simulink model "speedgoat_IO397_RCP"  (R2022b)
settings: Solver=FixedStepDiscrete  StartTime=0.0  StopTime=inf  RelTol=1e-3
PreLoadFcn:
  | Ts = 0.001;
  | FPGA_Frequency = 75000000;
undefined symbols (not defined in the file): IO397
libraries: speedgoatlib_fpga_dio x2, speedgoatlib_fpga_analog_io x2, speedgoatlib_fpga_inta x1, simulink x1, speedgoatlib_interrupt x1, speedgoatlib_fpga_pwm x1, speedgoatlib_fpga_quadrature x1, speedgoatlib_fpga x1
settings Model: SimulationMode=external  Creator=simon.beck  LastModifiedBy=jeffrey.gruenig
settings SolverCC: ConcurrentTasks=on  PositivePriorityOrder=on  MaxZcPerStep=1
settings DataIOCC: SaveFormat=StructureWithTime
settings OptimizationCC: BlockReduction=off  OptimizeBlockIOStorage=off  BufferReuse=off
settings DebuggingCC: UnderspecifiedInitializationDetection=Classic  MergeDetectMultiDrivingBlocksExec=none  TasksWithSamePriorityMsg=none
settings HardwareCC: ProdBitPerLong=64  ProdLongLongMode=on  ProdHWDeviceType=Intel->x86-64 (Linux 64)
settings ModelReferenceCC: EnableRefExpFcnMdlSchedulingChecks=on  PropagateSignalLabelsOutOfModel=off
settings RTWCC: Description=Simulink Real-Time  SystemTargetFile=slrealtime.tlc  TemplateMakefile=slrealtime_default_tmf  Toolchain=Simulink Real-Time Toolchain  BuildConfiguration=Faster Runs  CodeExecutionProfiling=on  TargetLang=C++  DLArmComputeVersion=19.05

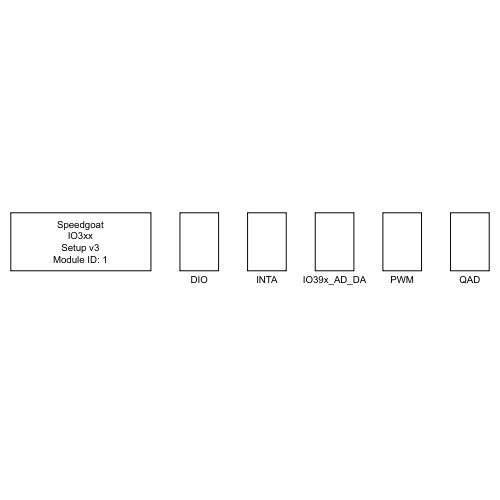
[thumbnail: Simulink's stored preview of the top-level diagram]
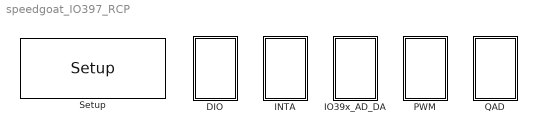
== system speedgoat_IO397_RCP ==
  DIO : Subsystem
  INTA : Subsystem
  IO39x_AD_DA : Subsystem
  PWM : Subsystem
  QAD : Subsystem
  Setup : speedgoatlib_fpga/Setup/Setup  board=IO397-50k  id=1  device_id=1  frontIO=None  rearIO=None  bitstreamFile=speedgoat_IO397_RCP.mat  rev=6.100000  timestamp_string=06/12/23 16:45:41  fpgaFreq=75 MHz  fpgaTick=13.33 ns  ProgSpiFlash=off  ProgBPIFlash=off  pciSlot=-1  useFpgaDmaController=off  PullRPort0=pull-up 3.3V  VioPort0=3.3V  PullRPort1=pull-up 3.3V  VioPort1=3.3V  PullRPort2=pull-up 3.3V  VioPort2=3.3V  PullRPort3=pull-up 3.3V  VioPort3=3.3V  PullRPort4=pull-up 3.3V  VioPort4=3.3V  PullRPort5=pull-up 3.3V  VioPort5=3.3V  PullRPort6=pull-up 3.3V  VioPort6=3.3V  diffLineTermination_rear1=on  diffLineTermination_rear2=on  diffLineTermination_rear3=on  diffLineTermination_rear4=on  diffLineTermination_rear5=on  diffLineTermination_rear6=on  diffLineTermination_rear7=on  diffLineTermination_rear8=on  PullRPort15=pull-up 3.3V  PullRPort31=pull-up 3.3V  PullRPort47=pull-up 3.3V  PullRPort63=pull-up 3.3V  diffLineTermination_1=on  diffLineTermination_2=on  diffLineTermination_3=on  diffLineTermination_4=on  diffLineTermination_5=on  diffLineTermination_6=on  diffLineTermination_7=on  diffLineTermination_8=on  diffLineTermination_9=on  diffLineTermination_10=on  diffLineTermination_11=on  diffLineTermination_12=on  diffLineTermination_13=on  diffLineTermination_14=on  diffLineTermination_15=on  diffLineTermination_16=on  diffLineTermination_17=on  diffLineTermination_18=on  diffLineTermination_19=on  diffLineTermination_20=on  diffLineTermination_21=on  diffLineTermination_22=on  diffLineTermination_23=on  diffLineTermination_24=on  diffLineTermination_25=on  diffLineTermination_26=on  diffLineTermination_27=on  diffLineTermination_28=on  diffLineTermination_29=on  diffLineTermination_30=on  diffLineTermination_31=on  diffLineTermination_32=on  Vo_36x_1=3.3V  Vi_Pull_36x_1=Floating  Vo_36x_2=3.3V  Vi_Pull_36x_2=Floating  Vo_36x_3=3.3V  Vi_Pull_36x_3=Floating  Vo_36x_4=3.3V  Vi_Pull_36x_4=Floating  Vo_36x_5=3.3V  Vi_Pull_36x_5=Floating  Vo_36x_6=3.3V  Vi_Pull_36x_6=Floating  Vo_36x_7=3.3V  Vi_Pull_36x_7=Floating  Vo_36x_8=3.3V  Vi_Pull_36x_8=Floating  Vo_36x_9_16=3.3V  Vi_Pull_36x_9_16=Floating  Vo_36x_17_24=3.3V  Vi_Pull_36x_17_24=Floating  Vo_36x_25_32=3.3V  Vi_Pull_36x_25_32=Floating  Vo_36x_33_40=3.3V  Vi_Pull_36x_33_40=Floating  Vo_36x_41_48=3.3V  Vi_Pull_36x_41_48=Floating  Vo_36x_49_56=3.3V  Vi_Pull_36x_49_56=Floating  Vo_36x_57_64=3.3V  Vi_Pull_36x_57_64=Floating
      settings: SourceProductName=Simulink Real-Time: Speedgoat I/O Blockset

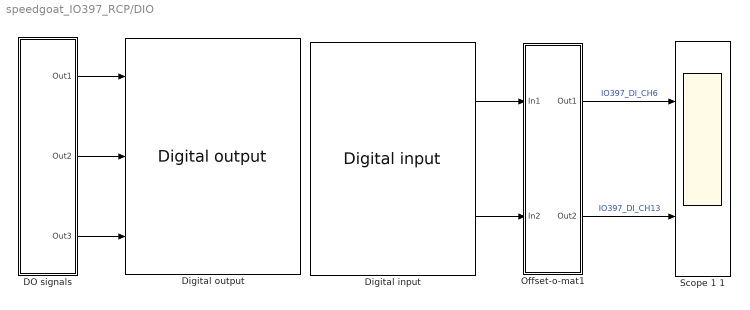
== system speedgoat_IO397_RCP/DIO ==
  DO signals : Subsystem
  Digital input : speedgoatlib_fpga_dio/Digital input  id=1  chan=[6,13]  ts=Ts  vectorizeOutput=off
      settings: SourceProductName=Simulink Real-Time: Speedgoat I/O Blockset
  Digital output : speedgoatlib_fpga_dio/Digital output  id=1  chan=[4,11,12]  init=[0]  reset=[0]  ts=Ts  vectorizeInput=off
      settings: SourceProductName=Simulink Real-Time: Speedgoat I/O Blockset
  Offset-o-mat1 : Subsystem
  Scope 1 1 : Scope  NumInputPorts=2
  wires:
  Offset-o-mat1/2(Out2) -> Scope 1 1/2  "IO397_DI_CH13"
  Offset-o-mat1/1(Out1) -> Scope 1 1/1  "IO397_DI_CH6"
  Digital input/2 -> Offset-o-mat1/2(In2)
  Digital input/1 -> Offset-o-mat1/1(In1)
  DO signals/3(Out3) -> Digital output/3
  DO signals/2(Out2) -> Digital output/2
  DO signals/1(Out1) -> Digital output/1

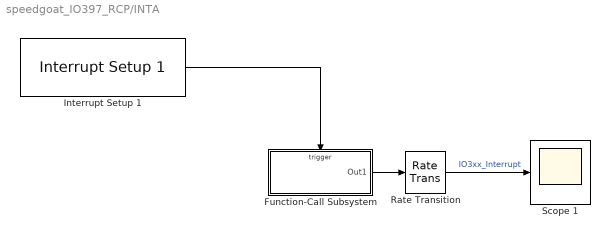
== system speedgoat_IO397_RCP/INTA ==
  Function-Call Subsystem : Subsystem  TreatAsAtomicUnit=on
  Interrupt Setup 1 : speedgoatlib_interrupt/Interrupt Setup 1  parModuleTrigger=off  parPollingMode=off  parPriorityConf=High  parPriority=241  confStartFcn=IO397_50k_start_public  confStopFcn=IO397_50k_stop_public  confIsrFcn=IO397_50k_isr_public  confMapFcn=IO397_50k_map_public  confHookFile=io397_50k_int_hooks.c  confIrqNr=-1  confIsPolling=off  confModID=16776961  confSelectedInt=Speedgoat IO397-50k interrupt  confSelectedId=1  confSelectedChannel=[]
  Rate Transition : RateTransition  Integrity=off
  "Scope 1 " : Scope
  wires:
  Rate Transition/1 -> "Scope 1 "/1  "IO3xx_Interrupt"
  Function-Call Subsystem/1(Out1) -> Rate Transition/1
  Interrupt Setup 1/1 -> Function-Call Subsystem/Trigger

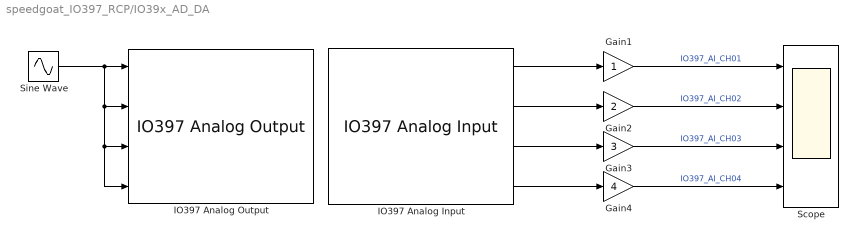
== system speedgoat_IO397_RCP/IO39x_AD_DA ==
  Gain1 : Gain
  Gain2 : Gain  Gain=2
  Gain3 : Gain  Gain=3
  Gain4 : Gain  Gain=4
  IO397 Analog Input : speedgoatlib_fpga_analog_io/IO397 Analog Input  openMaskCallback=0  id=1  chan=[1:4]  range=+-5 V  parAiTriggerMode=I/O Module Clock  parAiInternalSignal=None  parAiDioTriggerChannel=1  parAiSampleRate=0  trigger=Initiator  ts=0.001
      settings: SourceProductName=Simulink Real-Time: Speedgoat I/O Blockset
  IO397 Analog Output : speedgoatlib_fpga_analog_io/IO397 Analog Output  id=1  chan=1:4  initVal=0  resetVal=0  ts=0.001  span=+-5 V
      settings: SourceProductName=Simulink Real-Time: Speedgoat I/O Blockset
  Scope : Scope  NumInputPorts=4
  Sine Wave : Sin  Frequency=2*pi*(1/Ts)/50  SampleTime=Ts
  wires:
  IO397 Analog Input/4 -> Gain4/1
  IO397 Analog Input/3 -> Gain3/1
  IO397 Analog Input/2 -> Gain2/1
  IO397 Analog Input/1 -> Gain1/1
  Gain4/1 -> Scope/4  "IO397_AI_CH04"
  Gain3/1 -> Scope/3  "IO397_AI_CH03"
  Gain2/1 -> Scope/2  "IO397_AI_CH02"
  Gain1/1 -> Scope/1  "IO397_AI_CH01"
  Sine Wave/1 -> IO397 Analog Output/1, IO397 Analog Output/3, IO397 Analog Output/4, IO397 Analog Output/2

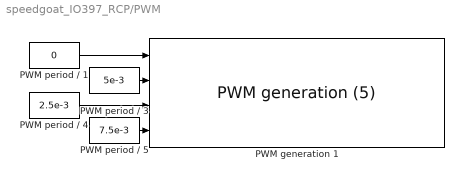
== system speedgoat_IO397_RCP/PWM ==
  PWM generation 1 : speedgoatlib_fpga_pwm/PWM generation (5)  id=1  chan=1  board=IO397-50k  ts=Ts  enableDma=off  pciSlot=[-1,-1]  delay=0  symmetric=Asymmetric - On and Off are freely configurable  b_is_complement_of_a=Independent of PWM A output  deadband=[0.0]  period=[10e-3]  frequency=100  ticks=749999  a_on=[0]  a_off=[0.0005]  pwm_a_dc=[0.0]  b_on=[0.00025]  b_off=[0.00075]  pwm_b_dc=[0]  c_on=[0.0]  c_off=[0.0]  protection=Disabled: A and B can be high at the same moment  enable_latch_half_period=off  pwm_update=At period starts  bit_width_pwm_gen=24  trigger_duration=[100e-6]  trigger_period_start=on  trigger_half_of_the_period=off  trigger_a_on=off  trigger_a_off=off  trigger_b_on=off  trigger_b_off=off  show_a_input=on  show_b_input=on  show_c_input=off  show_period_input=off  show_force_stop_input=off  idle_a=Low when PWM generation is halted  idle_b=Low when PWM generation is halted  idle_c=Low when PWM generation is halted  cancels_pwm_generation=on  invert_a=off  invert_b=off  invert_c=off
      settings: SourceProductName=Simulink Real-Time: Speedgoat I/O Blockset
  PWM period / 1 : Constant  Value=0
  PWM period / 3 : Constant  Value=5e-3
  PWM period / 4 : Constant  Value=2.5e-3
  PWM period / 5 : Constant  Value=7.5e-3
  wires:
  PWM period / 5/1 -> PWM generation 1/4
  PWM period / 3/1 -> PWM generation 1/2
  PWM period / 4/1 -> PWM generation 1/3
  PWM period / 1/1 -> PWM generation 1/1

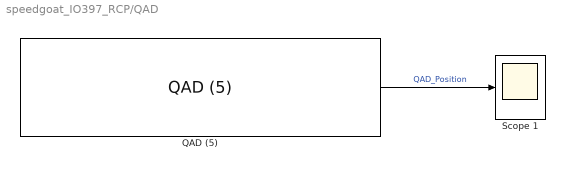
== system speedgoat_IO397_RCP/QAD ==
  QAD (5) : speedgoatlib_fpga_quadrature/QAD (5)  id=1  chan=[1]  sampleTime=Ts  enableDma=on  numOfSlots=[16]  sensorType=Capture A + B Signal  interpolatePosition=off  swapAB=off  indexControlMode=Ignore Index  latchMode=Disabled  gateIndex=No Gating  speedFilterWidth=4  showInputSpeedFilterWidth=off  glitchFilterSeconds=106.7e-9  glitchFilterSecondsEff=106.7e-9  showInputClearPosition=off  showInputClearIndexFound=off  showOutputPosition=on  showOutputTurn=off  showOutputSpeed=off  showOutputIndexFound=off  showOutputLastPulse=off
      settings: SourceProductName=Simulink Real-Time: Speedgoat I/O Blockset
  "Scope 1 " : Scope
  wires:
  QAD (5)/1 -> "Scope 1 "/1  "QAD_Position"

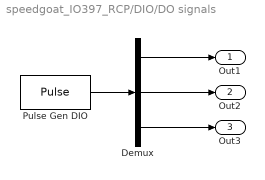
== system speedgoat_IO397_RCP/DIO/DO signals ==
  Demux : Demux  Outputs=3
  Pulse Gen DIO : DiscretePulseGenerator  Period=20  PulseWidth=[5,10,15]  SampleTime=Ts  VectorParams1D=off
  Out1 : Outport  VectorParamsAs1DForOutWhenUnconnected=off
  Out2 : Outport  Port=2  VectorParamsAs1DForOutWhenUnconnected=off
  Out3 : Outport  Port=3  VectorParamsAs1DForOutWhenUnconnected=off
  wires:
  Demux/1 -> Out1/1
  Demux/2 -> Out2/1
  Demux/3 -> Out3/1
  Pulse Gen DIO/1 -> Demux/1

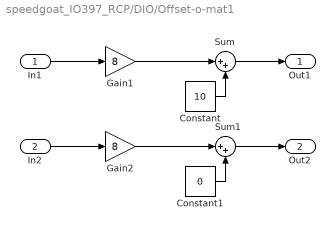
== system speedgoat_IO397_RCP/DIO/Offset-o-mat1 ==
  In1 : Inport
  In2 : Inport  Port=2
  Constant : Constant  Value=10
  Constant1 : Constant  Value=0
  Gain1 : Gain  Gain=8
  Gain2 : Gain  Gain=8
  Sum : Sum  Inputs=|++
  Sum1 : Sum  Inputs=|++
  Out1 : Outport  VectorParamsAs1DForOutWhenUnconnected=off
  Out2 : Outport  Port=2  VectorParamsAs1DForOutWhenUnconnected=off
  wires:
  Sum1/1 -> Out2/1
  Sum/1 -> Out1/1
  Constant/1 -> Sum/2
  In1/1 -> Gain1/1
  Constant1/1 -> Sum1/2
  In2/1 -> Gain2/1
  Gain1/1 -> Sum/1
  Gain2/1 -> Sum1/1

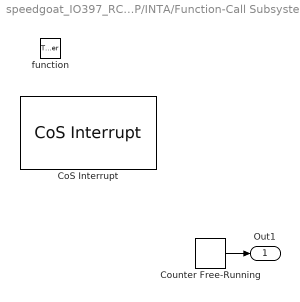
== system speedgoat_IO397_RCP/INTA/Function-Call Subsystem ==
  function : TriggerPort  TriggerType=function-call  VariantControl=Variant
  CoS Interrupt : speedgoatlib_fpga_inta/CoS Interrupt  id=1  ts=-1  debounce=0  delay=0  polarity=1
      settings: SourceProductName=Simulink Real-Time: Speedgoat I/O Blockset
  Counter Free-Running : simulink/Sources/Counter Free-Running  NumBits=32  tsamp=-1
  Out1 : Outport  InitialOutput=[0]  VectorParamsAs1DForOutWhenUnconnected=off
  wires:
  Counter Free-Running/1 -> Out1/1
